simulink model "TestGroup_v2"  (R2024b)
settings: Solver=VariableStepAuto  StartTime=0.0  StopTime=45  RelTol=1e-3
values from neighbouring files (symbols this model uses):
  K_altitude = lqr(A_altitude, B_altitude, Q_altitude, R_altitude)    [STATE_SPACE_CALCULATIONS.m]
undefined symbols (not defined in the file or in its folder): A_altitude, B_altitude
settings Model: Creator=hazza  LastModifiedBy=hazza

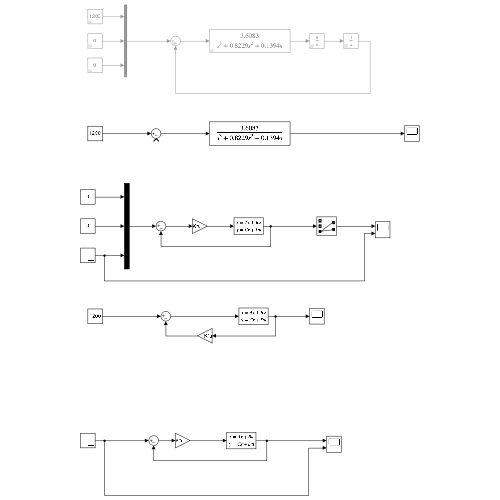
[thumbnail: Simulink's stored preview of the top-level diagram]
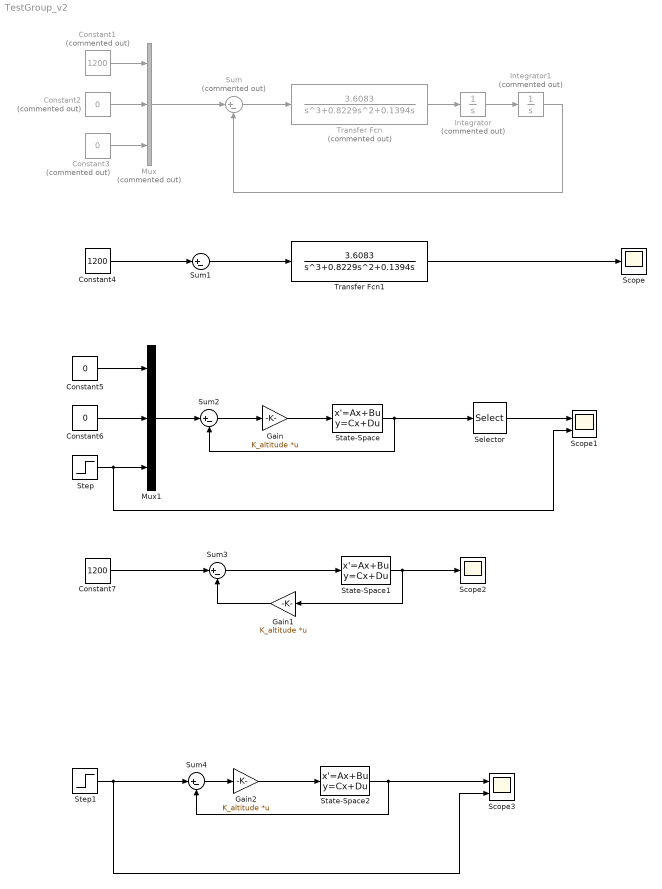
== system TestGroup_v2 ==
  Constant1 : Constant  Commented=on  Value=1200
  Constant2 : Constant  Commented=on  Value=0
  Constant3 : Constant  Commented=on  Value=0
  Constant4 : Constant  Value=1200
  Constant5 : Constant  Value=0
  Constant6 : Constant  Value=0
  Constant7 : Constant  Value=1200
  Gain : Gain  Gain=K_altitude  Multiplication=Matrix(K*u)
  Gain1 : Gain  Gain=K_altitude  Multiplication=Matrix(K*u)
  Gain2 : Gain  Gain=K_altitude  Multiplication=Matrix(K*u)
  Integrator : Integrator  Commented=on
  Integrator1 : Integrator  Commented=on
  Mux : Mux  Commented=on  Inputs=3
  Mux1 : Mux  Inputs=3
  Scope : Scope
  Scope1 : Scope  NumInputPorts=2
  Scope2 : Scope
  Scope3 : Scope  NumInputPorts=2
  Selector : Selector  InputPortWidth=3  IndexOptions=Index vector (dialog)  Indices=[3 3]  OutputSizes=1
  State-Space : StateSpace  A=A_altitude  B=B_altitude  C=[1 0 0; 0 1 0; 0 0 1]  D=[0; 0; 0]  InitialCondition=[0, 0, 1000]
  State-Space1 : StateSpace  A=A_altitude  B=B_altitude  C=[1 0 0; 0 1 0; 0 0 1]  D=[0; 0; 0]  InitialCondition=[1200, 0,0 ]
  State-Space2 : StateSpace  A=A_altitude  B=B_altitude  C=[1 0 0; 0 1 0; 0 0 1]  D=[0; 0; 0]  InitialCondition=[0, 0, 1500]
  Step : Step  Time=5  Before=1500  After=1200  SampleTime=0
  Step1 : Step  Time=5  Before=1500  After=1200  SampleTime=0
  Sum : Sum  Commented=on  Inputs=|+-
  Sum{1..4} (4 alike) : Sum  Inputs=|+-
  Transfer Fcn : TransferFcn  Commented=on  Numerator=3.6083  Denominator=[1, 0.8229, 0.1394, 0]
  Transfer Fcn1 : TransferFcn  Numerator=3.6083  Denominator=[1, 0.8229, 0.1394, 0]
  wires:
  Constant4/1 -> Sum1/1
  Transfer Fcn1/1 -> Scope/1
  Constant2/1 -> Mux/2
  Integrator/1 -> Integrator1/1
  Mux/1 -> Sum/1
  Integrator1/1 -> Sum/2
  Constant7/1 -> Sum3/1
  Sum1/1 -> Transfer Fcn1/1
  Mux1/1 -> Sum2/1
  Constant1/1 -> Mux/1
  Sum/1 -> Transfer Fcn/1
  State-Space1/1 -> Gain1/1, Scope2/1
  Gain/1 -> State-Space/1
  Sum3/1 -> State-Space1/1
  Gain1/1 -> Sum3/2
  State-Space/1 -> Sum2/2, Selector/1
  Sum2/1 -> Gain/1
  Constant3/1 -> Mux/3
  Transfer Fcn/1 -> Integrator/1
  Constant5/1 -> Mux1/1
  Constant6/1 -> Mux1/2
  Step/1 -> Scope1/2, Mux1/3
  Step1/1 -> Sum4/1, Scope3/2
  State-Space2/1 -> Sum4/2, Scope3/1
  Sum4/1 -> Gain2/1
  Gain2/1 -> State-Space2/1
  Selector/1 -> Scope1/1
